simulink model "demodulateur_c"  (R2021a)
settings: Solver=VariableStepAuto  StartTime=0.0  StopTime=10.0  RelTol=1e-3
libraries: dsparch4 x1, dspsrcs4 x1
settings Model: Creator=jimmypan  LastModifiedBy=jimmypan

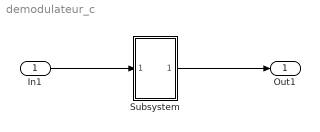
== system demodulateur_c ==
  In1 : Inport
  Subsystem : Subsystem
  Out1 : Outport
  wires:
  In1/1 -> Subsystem/1(In1)
  Subsystem/1(Out1) -> Out1/1

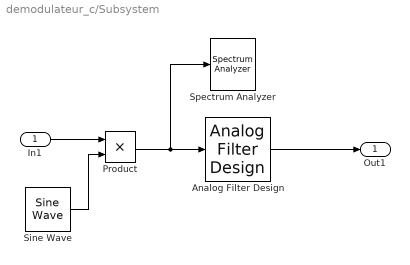
== system demodulateur_c/Subsystem ==
  In1 : Inport
  Analog Filter Design : dsparch4/Analog Filter Design  method=Butterworth  filttype=Lowpass  N=8  Wlo=130000  Whi=80  Rp=2  Rs=40
  Product : Product
  Sine Wave : dspsrcs4/Sine Wave  Amplitude=1  Frequency=500  Phase=0  SampleMode=Discrete  OutComplex=Real  CompMethod=Trigonometric fcn  TableSize=Speed  SampleTime=1/1000000  SamplesPerFrame=1  ResetState=Restart at time zero  OutputFrames=off  dataType=double  wordLen=16  udDataType=sfix(16)  fracBitsMode=Best precision  numFracBits=15  OutDataTypeStr=double  LastOutDataTypeStr=double
  Spectrum Analyzer : SpectrumAnalyzer
  Out1 : Outport
  wires:
  Sine Wave/1 -> Product/2
  In1/1 -> Product/1
  Analog Filter Design/1 -> Out1/1
  Product/1 -> Spectrum Analyzer/1, Analog Filter Design/1
